simulink model "GlideslopeController_model"  (R2020b)
settings: Solver=VariableStepAuto  StartTime=0.0  StopTime=10.0  RelTol=1e-3
values from neighbouring files (symbols this model uses):
  A_red_lo = sel(A_longitude_lo,1:5,1:5)    [GlideslopeController.m]
  B_red_lo = sel(A_longitude_lo,1:5,[6,7])    [GlideslopeController.m]
  C_red_lo = eye(5)    [GlideslopeController.m]
  D_red_lo = sel(D_longitude_lo,1:5,1:2)    [GlideslopeController.m]
undefined symbols (not defined in the file or in its folder): trim_control_lo, trim_thrust_lo
libraries: simulink_extras x2
settings Model: Creator=viran  LastModifiedBy=viran

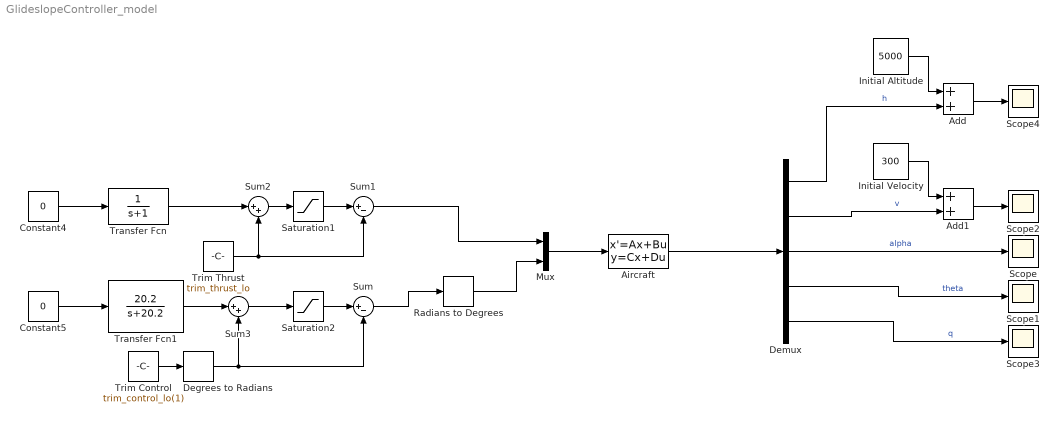
== system GlideslopeController_model ==
  Add : Sum
  Add1 : Sum
  Aircraft : StateSpace  A=A_red_lo  B=B_red_lo  C=C_red_lo  D=D_red_lo  InitialCondition=0
  Constant4 : Constant  Value=0
  Constant5 : Constant  Value=0
  Degrees to Radians : simulink_extras/Transformations/Degrees to Radians
  Demux : Demux  Outputs=5
  Initial Altitude : Constant  Value=5000
  Initial Velocity : Constant  Value=300
  Mux : Mux  Inputs=2
  Radians to Degrees : simulink_extras/Transformations/Radians to Degrees
  Saturation1 : Saturate  UpperLimit=19000  LowerLimit=1000
  Saturation2 : Saturate  UpperLimit=25*pi/180  LowerLimit=-25*pi/180
  Scope{,1..4} (5 alike) : Scope
  Sum : Sum  Inputs=|+-
  Sum1 : Sum  Inputs=|+-
  Sum2 : Sum  Inputs=|++
  Sum3 : Sum  Inputs=|++
  Transfer Fcn : TransferFcn  Denominator=[1 1]
  Transfer Fcn1 : TransferFcn  Numerator=[20.2]  Denominator=[1 20.2]
  Trim Control : Constant  Value=trim_control_lo(1)
  Trim Thrust : Constant  Value=trim_thrust_lo
  wires:
  Mux/1 -> Aircraft/1
  Sum1/1 -> Mux/1
  Aircraft/1 -> Demux/1
  Demux/3 -> Scope/1  "alpha"
  Demux/4 -> Scope1/1  "theta"
  Demux/5 -> Scope3/1  "q"
  Saturation1/1 -> Sum1/1
  Saturation2/1 -> Sum/1
  Trim Thrust/1 -> Sum1/2, Sum2/2
  Sum3/1 -> Saturation2/1
  Transfer Fcn1/1 -> Sum3/1
  Sum2/1 -> Saturation1/1
  Transfer Fcn/1 -> Sum2/1
  Trim Control/1 -> Degrees to Radians/1
  Degrees to Radians/1 -> Sum/2, Sum3/2
  Sum/1 -> Radians to Degrees/1
  Radians to Degrees/1 -> Mux/2
  Constant4/1 -> Transfer Fcn/1
  Constant5/1 -> Transfer Fcn1/1
  Demux/1 -> Add/2  "h"
  Initial Altitude/1 -> Add/1
  Add/1 -> Scope4/1
  Initial Velocity/1 -> Add1/1
  Demux/2 -> Add1/2  "v"
  Add1/1 -> Scope2/1
